simulink model "Model"  (R2018a)
settings: Solver=VariableStepAuto  StartTime=0.0  StopTime=inf  RelTol=1e-3
libraries: realtime_pacer_lib x1
settings Model: Creator=svenman  LastModifiedBy=Colin
settings CodeAppCC: StateflowObjectComments=on

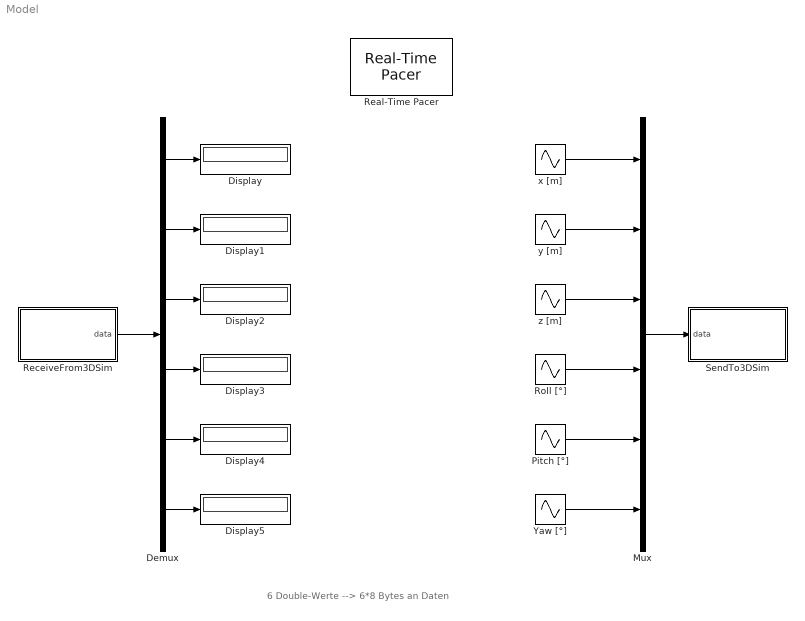
== system Model ==
  note: 6 Double-Werte --> 6*8 Bytes an Daten
  Demux : Demux  Outputs=6
  Display{,1..5} (6 alike) : Display
  Mux : Mux  Inputs=6
  Pitch [°] : Sin  Amplitude=45  Frequency=2*pi*1
  Real-Time Pacer : realtime_pacer_lib/Real-Time Pacer  simTimePerRealTime=1
  ReceiveFrom3DSim : Subsystem
  Roll [°] : Sin  Amplitude=2500  Bias=3100  Frequency=2*pi*1/20
  SendTo3DSim : Subsystem  TreatAsAtomicUnit=on  SystemSampleTime=0.01
  Yaw [°] : Sin  Amplitude=45  Frequency=2*pi*1
  x [m] : Sin  Amplitude=6  Frequency=2*pi*0.1
  y [m] : Sin  Amplitude=6  Frequency=2*pi*0.1  Phase=-pi/2
  z [m] : Sin  Amplitude=3  Bias=5  Frequency=2*pi*0.1
  wires:
  x [m]/1 -> Mux/1
  Yaw [°]/1 -> Mux/6
  y [m]/1 -> Mux/2
  z [m]/1 -> Mux/3
  Mux/1 -> SendTo3DSim/1(data)
  Roll [°]/1 -> Mux/4
  Pitch [°]/1 -> Mux/5
  ReceiveFrom3DSim/1(data) -> Demux/1
  Demux/1 -> Display/1
  Demux/2 -> Display1/1
  Demux/3 -> Display2/1
  Demux/4 -> Display3/1
  Demux/5 -> Display4/1
  Demux/6 -> Display5/1

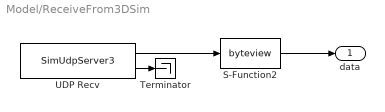
== system Model/ReceiveFrom3DSim ==
  S-Function2 : S-Function  FunctionName=byteview  Parameters=Ni,Ti,To  SFunctionDeploymentMode=off  EnableBusSupport=off  mask(Byte Viewer){Ni=6*8, Ti=uint8, To=double}
      mask prompts: Ni "Number of inputs (Ni)"; Ti "Input Type (Ti)"; To "Output Type (To)"
      mask help:
      | This block takes in input a vector of Ni signals belonging to a type Ti,
      |   puts them all in a contiguous memory zone, and reinterprets them as
      |   a vector of No signals belonging to a type To.
      |   The number of outputs No is equal to Ni*sizeof(To)/sizeof(Ti),
      |   where sizeof is the number of bytes of the type.
      mask Help:
      | This block takes in input a vector of Ni signals belonging to a type Ti,
      |   puts them all in a contiguous memory zone, and reinterprets them as
      |   a vector of No signals belonging to a type To.
      |   The number of outputs No is equal to Ni*sizeof(To)/sizeof(Ti),
      |   where sizeof is the number of bytes of the type.
      | 
      |   Typically you can use this block to decompose/recompose a double
      |   or a float into/from the bytes that composes it.
      mask TypeOptions Ti: double | single | int8 | uint8 | int16 | uint16 | int32 | uint32 | boolean
      mask TypeOptions To: double | single | int8 | uint8 | int16 | uint16 | int32 | uint32 | boolean
  Terminator : Terminator
  UDP Recv : S-Function  FunctionName=SimUdpServer3  Parameters=port,conn,bufsize,T  SFunctionDeploymentMode=off  EnableBusSupport=off  mask(UDP Receive){port=55556, conn=5, bufsize=6*8, T=-1}
      mask prompts: port "UDP Port"; conn "Maximum Number of Pending Connections"; bufsize "Buffer Size"; T "Sample Time"
      mask help:
      | This block receives bytes from an UDP/IP connection.
      |   The first output is a vector of data type uint8 (char), of size specifies
      |   as third parameter, containing the received bytes. The second output
      |   is a long integer containing the number of bytes that have actually been
      |   received during the last sample time interval,  (they could be less than the
      |   buffer size). If no bytes has been received, the last received ones
      |   are kept in the output. The first parameter is the UDP port number,
      |   and the second is the maximum number of pending connections.
      mask Help:
      | This block receives bytes from an UDP/IP connection.
      |   The first output is a vector of data type uint8 (char), of size specifies
      |   as third parameter, containing the received bytes. The second output
      |   is a long integer containing the number of bytes that have actually been
      |   received during the last sample time interval,  (they could be less than the
      |   buffer size). If no bytes has been received, the last received ones
      |   are kept in the output. The first parameter is the UDP port number,
      |   and the second is the maximum number of pending connections.
  data : Outport
  wires:
  UDP Recv/2 -> Terminator/1
  S-Function2/1 -> data/1
  UDP Recv/1 -> S-Function2/1

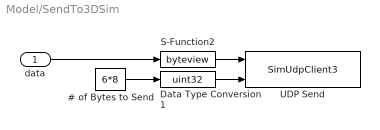
== system Model/SendTo3DSim ==
  data : Inport
  # of Bytes to Send : Constant  Value=6*8
  Data Type Conversion1 : DataTypeConversion  OutDataTypeStr=uint32  SaturateOnIntegerOverflow=on  RndMeth=Zero
  S-Function2 : S-Function  FunctionName=byteview  Parameters=Ni,Ti,To  SFunctionDeploymentMode=off  EnableBusSupport=off  mask(Byte Viewer){Ni=6, Ti=double, To=uint8}
      mask prompts: Ni "Number of inputs (Ni)"; Ti "Input Type (Ti)"; To "Output Type (To)"
      mask help:
      | This block takes in input a vector of Ni signals belonging to a type Ti,
      |   puts them all in a contiguous memory zone, and reinterprets them as
      |   a vector of No signals belonging to a type To.
      |   The number of outputs No is equal to Ni*sizeof(To)/sizeof(Ti),
      |   where sizeof is the number of bytes of the type.
      mask Help:
      | This block takes in input a vector of Ni signals belonging to a type Ti,
      |   puts them all in a contiguous memory zone, and reinterprets them as
      |   a vector of No signals belonging to a type To.
      |   The number of outputs No is equal to Ni*sizeof(To)/sizeof(Ti),
      |   where sizeof is the number of bytes of the type.
      | 
      |   Typically you can use this block to decompose/recompose a double
      |   or a float into/from the bytes that composes it.
      mask TypeOptions Ti: double | single | int8 | uint8 | int16 | uint16 | int32 | uint32 | boolean
      mask TypeOptions To: double | single | int8 | uint8 | int16 | uint16 | int32 | uint32 | boolean
  UDP Send : S-Function  FunctionName=SimUdpClient3  Parameters=host,port,bufsize,T  SFunctionDeploymentMode=off  EnableBusSupport=off  mask(UDP Send){host=127.0.0.1, port=55555, bufsize=6*8, T=-1}
      mask prompts: host "Host name"; port "UDP Port"; bufsize "Buffer Size"; T "Sample Time"
      mask help:
      | This block sends bytes to an host computer via UDP/IP.
      |   The first input is the vector of data type uint8 (char) containing the
      |   bytes to be sent. The size of the vector is specified with the third
      |   parameter. The second input is a long integer containing the number
      |   of bytes to be sent from the first input vector (they could be less than
      |   the buffer size). The first parameter is either the hostname or the IP
      |   address of the host computer where the data need to be sent.
      |   The second parameter is the UDP port number.
      mask Help:
      | This block sends bytes to an host computer via UDP/IP.
      |   The first input is the vector of data type uint8 (char) containing the
      |   bytes to be sent. The size of the vector is specified with the third
      |   parameter. The second input is a long integer containing the number
      |   of bytes to be sent from the first input vector (they could be less than
      |   the buffer size). The first parameter is either the hostname or the IP
      |   address of the host computer where the data need to be sent.
      |   The second parameter is the UDP port number.
  wires:
  S-Function2/1 -> UDP Send/1
  data/1 -> S-Function2/1
  # of Bytes to Send/1 -> Data Type Conversion1/1
  Data Type Conversion1/1 -> UDP Send/2
